simulink model "steady_state_error_type_1"  (R2018b)
settings: Solver=VariableStepAuto  StartTime=0.0  StopTime=100  RelTol=1e-3
model workspace (MAT data in the model file):
  A = Simulink.Parameter
  A.Value = 1
  A.DataType = 'auto'
  A.DocUnits = 'm^2'
  A.Dimensions = [1 1]
  h0 = Simulink.Parameter
  h0.Value = 0
  h0.DataType = 'auto'
  h0.DocUnits = '<m>'
  h0.Dimensions = [1 1]
  k1 = Simulink.Parameter
  k1.Value = 10
  k1.DataType = 'auto'
  k1.Dimensions = [1 1]
  qin = Simulink.Parameter
  qin.Value = 0.4
  qin.DataType = 'auto'
  qin.DocUnits = '<m^3/s>'
  qin.Dimensions = [1 1]
settings Model: OrderedModelArguments=off  Creator=waleed.elbadry  LastModifiedBy=waleed.elbadry

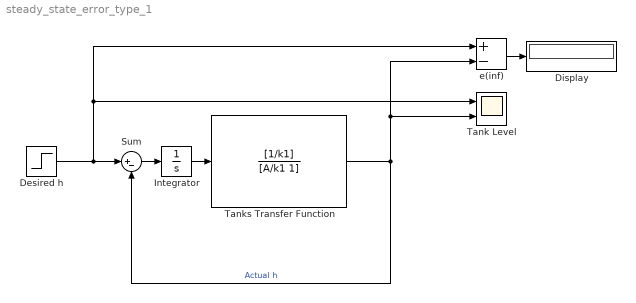
== system steady_state_error_type_1 ==
  Desired h : Step  Time=0  After=4  SampleTime=0
  Display : Display
      settings: Decimation=2
  Integrator : Integrator
  Sum : Sum  Inputs=|+-
  Tank Level : Scope  NumInputPorts=2
  Tanks Transfer Function : TransferFcn  Numerator=[1/k1]  Denominator=[A/k1 1]
  e(inf) : Sum  Inputs=+-
  wires:
  Tanks Transfer Function/1 -> e(inf)/2, Tank Level/2, Sum/2  "Actual h"
  Desired h/1 -> e(inf)/1, Tank Level/1, Sum/1
  e(inf)/1 -> Display/1
  Sum/1 -> Integrator/1
  Integrator/1 -> Tanks Transfer Function/1
